simulink model "TST_ASDrf_SelectParameter"  (R2016b)
settings: Solver=FixedStepDiscrete  StartTime=0.0  StopTime=simTime  FixedStep=sampleTime  RelTol=1e-3
values from neighbouring files (symbols this model uses):
  testCase = 1    [initTST_ASDrf_SelectParameter_001.m]
libraries: simulink x3, UnitTest_Lib x1
settings Model: Creator=zhengjinyan  LastModifiedBy=zhengjinyan
settings DebuggingCC: SignalRangeChecking=error

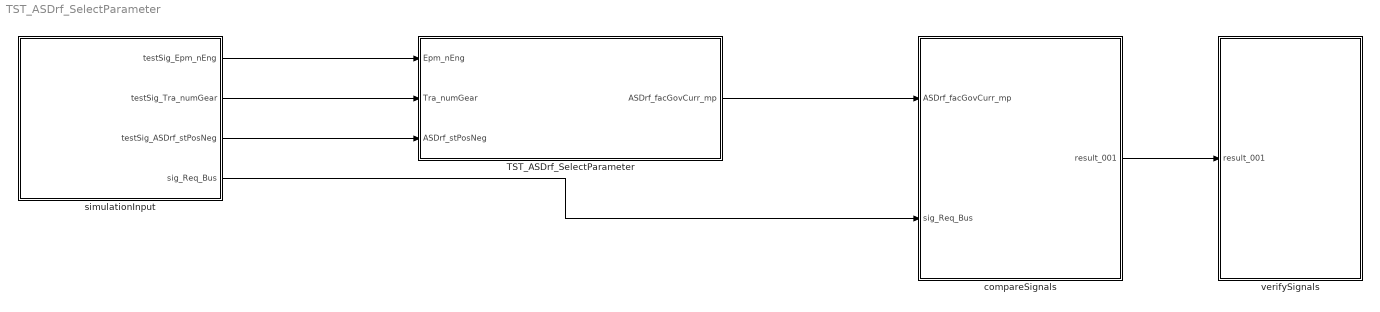
== system TST_ASDrf_SelectParameter ==
  TST_ASDrf_SelectParameter : Subsystem
  compareSignals : Subsystem
  simulationInput : Subsystem
  verifySignals : Subsystem
  wires:
  simulationInput/1(testSig_Epm_nEng) -> TST_ASDrf_SelectParameter/1(Epm_nEng)
  simulationInput/2(testSig_Tra_numGear) -> TST_ASDrf_SelectParameter/2(Tra_numGear)
  simulationInput/3(testSig_ASDrf_stPosNeg) -> TST_ASDrf_SelectParameter/3(ASDrf_stPosNeg)
  TST_ASDrf_SelectParameter/1(ASDrf_facGovCurr_mp) -> compareSignals/1(ASDrf_facGovCurr_mp)
  simulationInput/4(sig_Req_Bus) -> compareSignals/2(sig_Req_Bus)
  compareSignals/1(result_001) -> verifySignals/1(result_001)

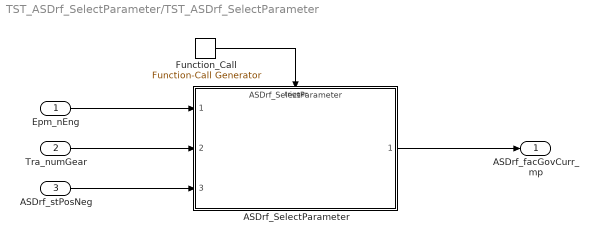
== system TST_ASDrf_SelectParameter/TST_ASDrf_SelectParameter ==
  Epm_nEng : Inport
  Tra_numGear : Inport  Port=2
  ASDrf_stPosNeg : Inport  Port=3
  ASDrf_SelectParameter : ModelReference  ModelNameDialog=ASDrf_SelectParameter  SimulationMode=Normal  ModelReferenceVersion=1.24  TriggerPortName=function  TriggerPortTriggerType=function-call  TriggerPortStatesWhenEnabling=held
  Function_Call : simulink/Ports & Subsystems/Function-Call Generator  sample_time=sampleTime  numberOfIterations=1
  ASDrf_facGovCurr_mp : Outport
  wires:
  Function_Call/1 -> ASDrf_SelectParameter/Trigger
  Epm_nEng/1 -> ASDrf_SelectParameter/1
  Tra_numGear/1 -> ASDrf_SelectParameter/2
  ASDrf_stPosNeg/1 -> ASDrf_SelectParameter/3
  ASDrf_SelectParameter/1 -> ASDrf_facGovCurr_mp/1

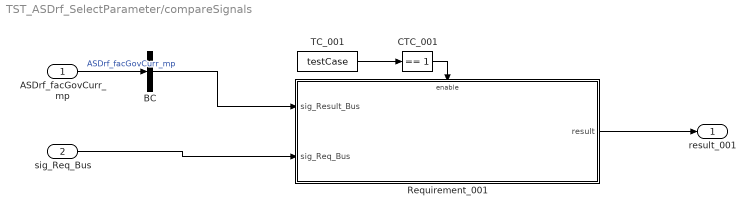
== system TST_ASDrf_SelectParameter/compareSignals ==
  ASDrf_facGovCurr_mp : Inport
  sig_Req_Bus : Inport  Port=2
  BC : BusCreator  Inputs=1
  CTC_001 : simulink/Logic and Bit Operations/Compare To Constant  relop===  const=1  OutDataTypeStr=boolean
  Requirement_001 : Subsystem
  TC_001 : Constant  Value=testCase
  result_001 : Outport
  wires:
  ASDrf_facGovCurr_mp/1 -> BC/1  "ASDrf_facGovCurr_mp"
  TC_001/1 -> CTC_001/1
  CTC_001/1 -> Requirement_001/Enable
  sig_Req_Bus/1 -> Requirement_001/2(sig_Req_Bus)
  BC/1 -> Requirement_001/1(sig_Result_Bus)
  Requirement_001/1(result) -> result_001/1

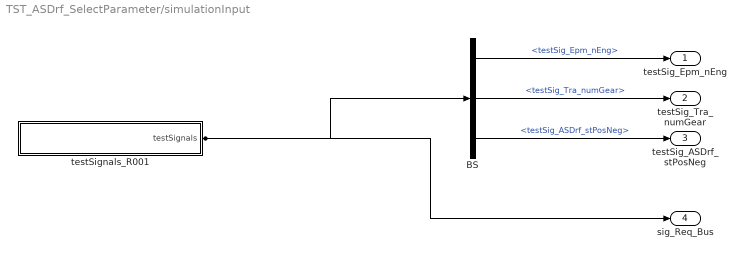
== system TST_ASDrf_SelectParameter/simulationInput ==
  BS : BusSelector  OutputSignals=testSig_Epm_nEng,testSig_Tra_numGear,testSig_ASDrf_stPosNeg
  testSignals_R001 : Subsystem
  testSig_Epm_nEng : Outport
  testSig_Tra_numGear : Outport  Port=2
  testSig_ASDrf_stPosNeg : Outport  Port=3
  sig_Req_Bus : Outport  Port=4
  wires:
  BS/1 -> testSig_Epm_nEng/1  "<testSig_Epm_nEng>"
  BS/2 -> testSig_Tra_numGear/1  "<testSig_Tra_numGear>"
  BS/3 -> testSig_ASDrf_stPosNeg/1  "<testSig_ASDrf_stPosNeg>"
  testSignals_R001/1(testSignals) -> BS/1, sig_Req_Bus/1

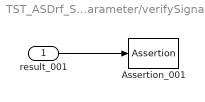
== system TST_ASDrf_SelectParameter/verifySignals ==
  result_001 : Inport
  Assertion_001 : Assertion  Enabled=off
  wires:
  result_001/1 -> Assertion_001/1

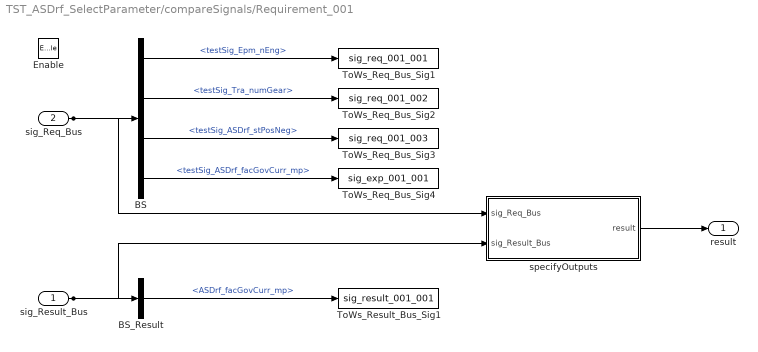
== system TST_ASDrf_SelectParameter/compareSignals/Requirement_001 ==
  sig_Result_Bus : Inport
  sig_Req_Bus : Inport  Port=2
  Enable : EnablePort
  BS : BusSelector  OutputSignals=testSig_Epm_nEng,testSig_Tra_numGear,testSig_ASDrf_stPosNeg,testSig_ASDrf_facGovCurr_mp
  BS_Result : BusSelector  OutputSignals=ASDrf_facGovCurr_mp
  ToWs_Req_Bus_Sig1 : ToWorkspace  VariableName=sig_req_001_001  SaveFormat=Structure With Time
  ToWs_Req_Bus_Sig2 : ToWorkspace  VariableName=sig_req_001_002  SaveFormat=Structure With Time
  ToWs_Req_Bus_Sig3 : ToWorkspace  VariableName=sig_req_001_003  SaveFormat=Structure With Time
  ToWs_Req_Bus_Sig4 : ToWorkspace  VariableName=sig_exp_001_001  SaveFormat=Structure With Time
  ToWs_Result_Bus_Sig1 : ToWorkspace  VariableName=sig_result_001_001  SaveFormat=Structure With Time
  specifyOutputs : Subsystem
  result : Outport
  wires:
  sig_Req_Bus/1 -> BS/1, specifyOutputs/1(sig_Req_Bus)
  BS/1 -> ToWs_Req_Bus_Sig1/1  "<testSig_Epm_nEng>"
  BS/2 -> ToWs_Req_Bus_Sig2/1  "<testSig_Tra_numGear>"
  BS/3 -> ToWs_Req_Bus_Sig3/1  "<testSig_ASDrf_stPosNeg>"
  BS/4 -> ToWs_Req_Bus_Sig4/1  "<testSig_ASDrf_facGovCurr_mp>"
  sig_Result_Bus/1 -> BS_Result/1, specifyOutputs/2(sig_Result_Bus)
  BS_Result/1 -> ToWs_Result_Bus_Sig1/1  "<ASDrf_facGovCurr_mp>"
  specifyOutputs/1(result) -> result/1

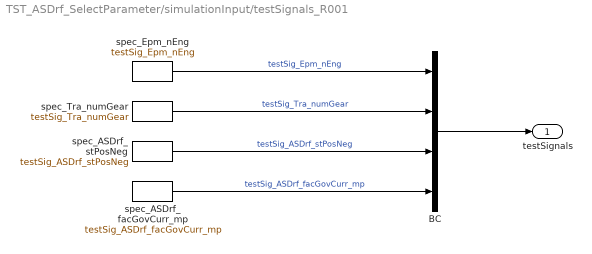
== system TST_ASDrf_SelectParameter/simulationInput/testSignals_R001 ==
  BC : BusCreator  Inputs=4
  spec_ASDrf_facGovCurr_mp : FromWorkspace  VariableName=testSig_ASDrf_facGovCurr_mp  Interpolate=off  OutputAfterFinalValue=Holding final value
  spec_ASDrf_stPosNeg : FromWorkspace  VariableName=testSig_ASDrf_stPosNeg  Interpolate=off  OutputAfterFinalValue=Holding final value
  spec_Epm_nEng : FromWorkspace  VariableName=testSig_Epm_nEng  Interpolate=off  OutputAfterFinalValue=Holding final value
  spec_Tra_numGear : FromWorkspace  VariableName=testSig_Tra_numGear  Interpolate=off  OutputAfterFinalValue=Holding final value
  testSignals : Outport
  wires:
  BC/1 -> testSignals/1
  spec_Epm_nEng/1 -> BC/1  "testSig_Epm_nEng"
  spec_Tra_numGear/1 -> BC/2  "testSig_Tra_numGear"
  spec_ASDrf_stPosNeg/1 -> BC/3  "testSig_ASDrf_stPosNeg"
  spec_ASDrf_facGovCurr_mp/1 -> BC/4  "testSig_ASDrf_facGovCurr_mp"

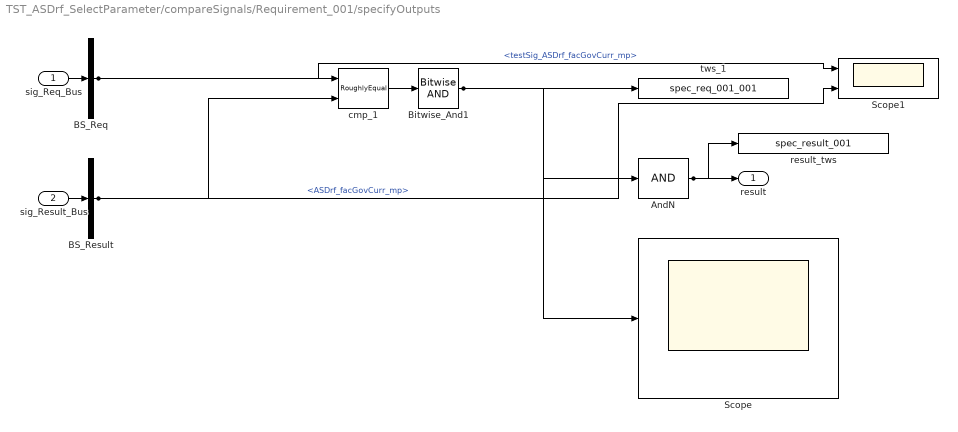
== system TST_ASDrf_SelectParameter/compareSignals/Requirement_001/specifyOutputs ==
  sig_Req_Bus : Inport
  sig_Result_Bus : Inport  Port=2
  AndN : Logic  Inputs=1
  BS_Req : BusSelector  OutputSignals=testSig_ASDrf_facGovCurr_mp
  BS_Result : BusSelector  OutputSignals=ASDrf_facGovCurr_mp
  Bitwise_And1 : simulink/Logic and Bit Operations/Bitwise Operator  logicop=AND  UseBitMask=off  BitMask=bin2dec('11011001')  BitMaskRealWorld=Stored Integer
  Scope : Scope
  Scope1 : Scope  NumInputPorts=2
  cmp_1 : UnitTest_Lib/RoughlyEqual  slope=0.1
  result_tws : ToWorkspace  VariableName=spec_result_001
  tws_1 : ToWorkspace  VariableName=spec_req_001_001
  result : Outport
  wires:
  sig_Req_Bus/1 -> BS_Req/1
  sig_Result_Bus/1 -> BS_Result/1
  AndN/1 -> result/1, result_tws/1
  BS_Req/1 -> cmp_1/1, Scope1/1  "<testSig_ASDrf_facGovCurr_mp>"
  BS_Result/1 -> cmp_1/2, Scope1/2  "<ASDrf_facGovCurr_mp>"
  cmp_1/1 -> Bitwise_And1/1
  Bitwise_And1/1 -> tws_1/1, AndN/1, Scope/1
